simulink model "pendulum"  (R2017b)
settings: Solver=VariableStepAuto  StartTime=0.0  StopTime=10.0  RelTol=1e-3
undefined symbols (not defined in the file): a_0, a_1, a_2, dfi_0, fi_0
settings Model: Creator=ASROCK  LastModifiedBy=ASROCK

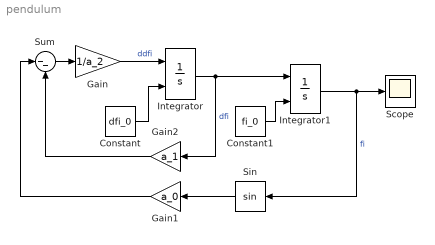
== system pendulum ==
  Constant : Constant  Value=dfi_0
  Constant1 : Constant  Value=fi_0
  Gain : Gain  Gain=1/a_2
  Gain1 : Gain  Gain=a_0
  Gain2 : Gain  Gain=a_1
  Integrator : Integrator  InitialConditionSource=external
  Integrator1 : Integrator  InitialConditionSource=external
  Scope : Scope
  Sin : Trigonometry
  Sum : Sum  Inputs=|--
  wires:
  Integrator/1 -> Integrator1/1, Gain2/1  "dfi"
  Sum/1 -> Gain/1
  Gain/1 -> Integrator/1  "ddfi"
  Integrator1/1 -> Sin/1, Scope/1  "fi"
  Gain2/1 -> Sum/2
  Gain1/1 -> Sum/1
  Sin/1 -> Gain1/1
  Constant/1 -> Integrator/2
  Constant1/1 -> Integrator1/2
